simulink model "P_4_3_c_Eroforras"  (R2022b)
settings: Solver=VariableStepAuto  StartTime=0.0  StopTime=200  RelTol=1e-3
undefined symbols (not defined in the file or in its folder): m, n
libraries: dspstat3 x1
settings Model: Creator=csokam  LastModifiedBy=Mark
settings SolverCC: AlgebraicLoopSolver=TrustRegion
settings DebuggingCC: UnconnectedInputMsg=warning  UnconnectedOutputMsg=warning  UnconnectedLineMsg=warning  SFMachineParentedDataDiag=warning
settings ModelReferenceCC: EnableRefExpFcnMdlSchedulingChecks=on
settings RTWCC: DLArmComputeVersion=19.05

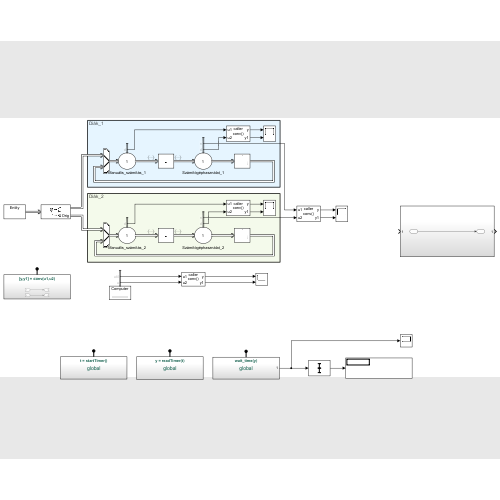
[thumbnail: Simulink's stored preview of the top-level diagram]
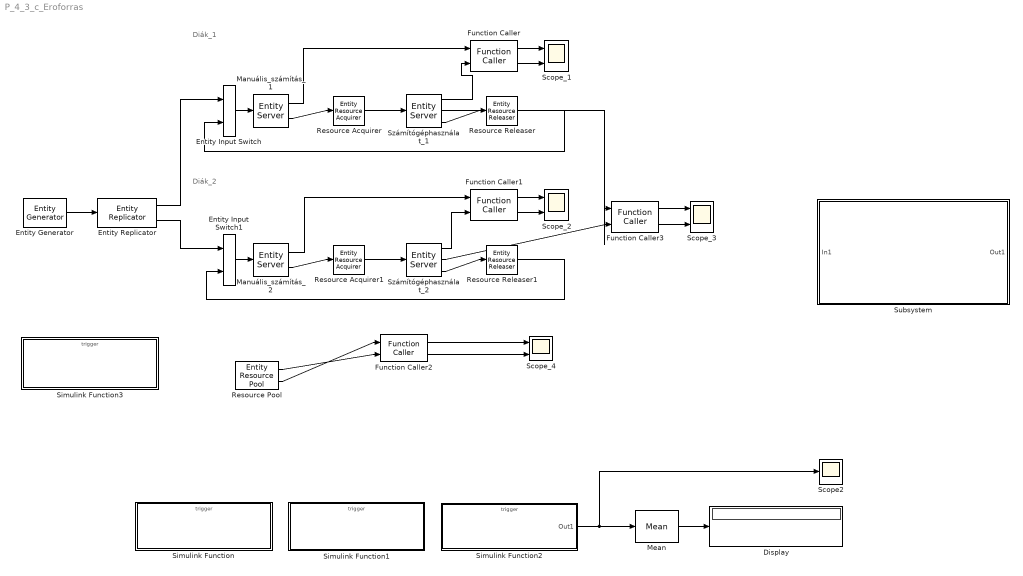
== system P_4_3_c_Eroforras ==
  note: Diák_2
  note: Diák_1
  Display : Display
      settings: Format=decimal (Stored Integer)
  Entity Input Switch : EntityInputSwitch  InputPortMessageModes=m,m  OutputPortMessageModes=m
  Entity Input Switch1 : EntityInputSwitch  InputPortMessageModes=m,m  OutputPortMessageModes=m
  Entity Generator : EntityGenerator  OutputPortMessageModes=m  TimeSource=MATLAB action  IntergenerationTimeAction=dt= inf;  AttributeName=Timer  EntityType=Structured  EntityTypeName=Entity
  Entity Replicator : EntityReplicator  InputPortMessageModes=m  OutputPortMessageModes=m,m
  Function Caller{,1..3} (4 alike) : FunctionCaller  FunctionPrototype=[y,y1] = conv(u1,u2)  InputArgumentSpecifications=<Enter example>  OutputArgumentSpecifications=<Enter example>
  Manuális_számítás_1 : EntityServer  InputPortMessageModes=m  OutputPortMessageModes=n,m  Capacity=1  ServiceTimeSource=MATLAB action  ServiceTimeAction=|  NumberEntitiesDeparted=on
      | persistent rngInit;
      | if isempty(rngInit)
      |     seed = 12345;
      |     rng(seed);
      |     rngInit = true;
      | end
      | 
      | % Pattern: Uniform distribution
      | % m: Minimum, M: Maximum
      | m = 20; M = 30;
      | dt = m + (M - m) * rand;
      settings: OutputPortMap=o0,o9
  Manuális_számítás_2 : EntityServer  InputPortMessageModes=m  OutputPortMessageModes=n,m  Capacity=1  ServiceTimeSource=MATLAB action  ServiceTimeAction=|  NumberEntitiesDeparted=on
      | persistent rngInit;
      | if isempty(rngInit)
      |     seed = 12345;
      |     rng(seed);
      |     rngInit = true;
      | end
      | 
      | % Pattern: Uniform distribution
      | % m: Minimum, M: Maximum
      | m = 15; M = 20;
      | dt = m + (M - m) * rand;
      settings: OutputPortMap=o0,o9
  Mean : dspstat3/Mean  run=off  InputProcessing=Columns as channels (frame based)  reset_popup=None  directionMode=Each column  dimension=1  roiEnable=off  roiType=Rectangles  roiPortion=Entire ROI  roiOutput=Individual statistics for each ROI  roiFlag=off  roundingMode=Floor  overflowMode=off  outputDataTypeStr=Inherit: Same as accumulator  outputMin=[]  outputMax=[]  outputLastDataTypeStr=Inherit: Same as accumulator
  Resource Acquirer : EntityResourceAcquirer  InputPortMessageModes=m  OutputPortMessageModes=m  EntryAction=entity.Timer = startTimer();  ExitAction=|  ResourceName=Computer
      | elapsedTime = readTimer(entity.Timer);
      | wait_time(elapsedTime);
      settings: OutputPortMap=o3
  Resource Acquirer1 : EntityResourceAcquirer  InputPortMessageModes=m  OutputPortMessageModes=m  EntryAction=entity.Timer= startTimer();  ExitAction=|  ResourceName=Computer
      | elapsedTime = readTimer(entity.Timer);
      | wait_time(elapsedTime);
      settings: OutputPortMap=o3
  Resource Releaser : EntityResourceReleaser  InputPortMessageModes=m  OutputPortMessageModes=m  ResourceToRelease=Selected  ResourceName=Computer
  Resource Releaser1 : EntityResourceReleaser  InputPortMessageModes=m  OutputPortMessageModes=m  ResourceToRelease=Selected  ResourceName=Computer
  Resource Pool : EntityResourcePool  ResourceName=Computer  ResourceAmount=1  AmountInUse=on  AverageUtilization=on
      settings: OutputPortMap=o0,o1
  Scope2 : Scope
  Scope_{1..4} (4 alike) : Scope  NumInputPorts=2
  Simulink Function : Subsystem  TreatAsAtomicUnit=on
  Simulink Function1 : Subsystem  TreatAsAtomicUnit=on
  Simulink Function2 : Subsystem  TreatAsAtomicUnit=on
  Simulink Function3 : Subsystem  TreatAsAtomicUnit=on
  Subsystem : Subsystem
  Számítógéphasználat_1 : EntityServer  InputPortMessageModes=m  OutputPortMessageModes=n,n,m  Capacity=1  ServiceTimeSource=MATLAB action  ServiceTimeAction=|  NumberEntitiesDeparted=on  NumberEntitiesInBlock=on
      | persistent rngInit;
      | if isempty(rngInit)
      |     seed = 12345;
      |     rng(seed);
      |     rngInit = true;
      | end
      | 
      | % Pattern: Uniform distribution
      | % m: Minimum, M: Maximum
      | m = 10; M = 15;
      | dt = m + (M - m) * rand;
      settings: OutputPortMap=o0,o1,o9
  Számítógéphasználat_2 : EntityServer  InputPortMessageModes=m  OutputPortMessageModes=n,n,m  Capacity=1  ServiceTimeSource=MATLAB action  ServiceTimeAction=|  NumberEntitiesDeparted=on  NumberEntitiesInBlock=on
      | persistent rngInit;
      | if isempty(rngInit)
      |     seed = 12345;
      |     rng(seed);
      |     rngInit = true;
      | end
      | 
      | % Pattern: Uniform distribution
      | % m: Minimum, M: Maximum
      | m = 5; M = 25;
      | dt = m + (M - m) * rand;
      settings: OutputPortMap=o0,o1,o9
  wires:
  Entity Generator/1 -> Entity Replicator/1
  Entity Replicator/1 -> Entity Input Switch/1
  Entity Input Switch/1 -> Manuális_számítás_1/1
  Manuális_számítás_1/2 -> Resource Acquirer/1
  Resource Acquirer/1 -> Számítógéphasználat_1/1
  Számítógéphasználat_1/3 -> Resource Releaser/1
  Resource Releaser/1 -> Entity Input Switch/2
  Manuális_számítás_1/1 -> Function Caller/1
  Számítógéphasználat_1/1 -> Function Caller/2
  Function Caller/1 -> Scope_1/1
  Function Caller/2 -> Scope_1/2
  Function Caller1/2 -> Scope_2/2
  Function Caller1/1 -> Scope_2/1
  Manuális_számítás_2/1 -> Function Caller1/1
  Manuális_számítás_2/2 -> Resource Acquirer1/1
  Entity Replicator/2 -> Entity Input Switch1/1
  Számítógéphasználat_2/1 -> Function Caller1/2
  Számítógéphasználat_2/3 -> Resource Releaser1/1
  Resource Acquirer1/1 -> Számítógéphasználat_2/1
  Entity Input Switch1/1 -> Manuális_számítás_2/1
  Resource Releaser1/1 -> Entity Input Switch1/2
  Resource Pool/1 -> Function Caller2/2
  Resource Pool/2 -> Function Caller2/1
  Function Caller2/1 -> Scope_4/1
  Function Caller2/2 -> Scope_4/2
  Számítógéphasználat_1/2 -> Function Caller3/1
  Számítógéphasználat_2/2 -> Function Caller3/2
  Function Caller3/1 -> Scope_3/1
  Function Caller3/2 -> Scope_3/2
  Simulink Function2/1(Out1) -> Mean/1, Scope2/1
  Mean/1 -> Display/1

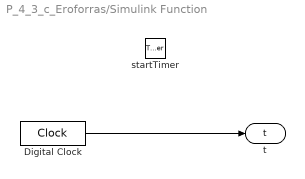
== system P_4_3_c_Eroforras/Simulink Function ==
  startTimer : TriggerPort  TriggerType=function-call  IsSimulinkFunction=on  FunctionName=startTimer  VariantControl=(inherit)
  Digital Clock : DigitalClock  SampleTime=-1
  t : ArgOut  DisableCoverage=on  ArgumentName=t
  wires:
  Digital Clock/1 -> t/1

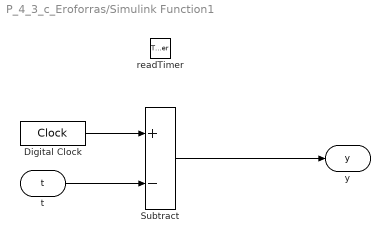
== system P_4_3_c_Eroforras/Simulink Function1 ==
  readTimer : TriggerPort  TriggerType=function-call  IsSimulinkFunction=on  FunctionName=readTimer  VariantControl=(inherit)
  Digital Clock : DigitalClock  SampleTime=-1
  Subtract : Sum  Inputs=+-
  t : ArgIn  ArgumentName=t
  y : ArgOut  ArgumentName=y
  wires:
  Digital Clock/1 -> Subtract/1
  t/1 -> Subtract/2
  Subtract/1 -> y/1

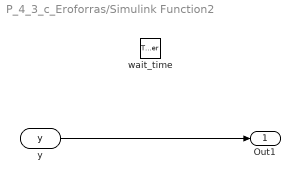
== system P_4_3_c_Eroforras/Simulink Function2 ==
  wait_time : TriggerPort  TriggerType=function-call  IsSimulinkFunction=on  FunctionName=wait_time  VariantControl=(inherit)
  y : ArgIn  DisableCoverage=on  ArgumentName=y
  Out1 : Outport  SourceOfInitialOutputValue=Input signal
  wires:
  y/1 -> Out1/1

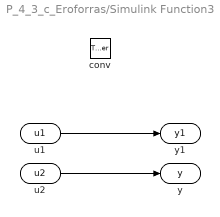
== system P_4_3_c_Eroforras/Simulink Function3 ==
  conv : TriggerPort  TriggerType=function-call  IsSimulinkFunction=on  FunctionName=conv  FunctionVisibility=scoped  VariantControl=(inherit)
  u1 : ArgIn  DisableCoverage=on  ArgumentName=u1
  u2 : ArgIn  Port=2  ArgumentName=u2
  y : ArgOut  DisableCoverage=on  ArgumentName=y
  y1 : ArgOut  Port=2  ArgumentName=y1
  wires:
  u1/1 -> y1/1
  u2/1 -> y/1

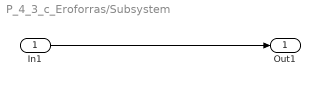
== system P_4_3_c_Eroforras/Subsystem ==
  In1 : Inport
  Out1 : Outport
  wires:
  In1/1 -> Out1/1
